simulink model "mekai_longitudinal_vehicle_starter"  (R2025b)
settings: Solver=ode45  StartTime=0.0  StopTime=simConfig.stopTime  RelTol=1e-3
undefined symbols (not defined in the file or in its folder): driver, params
settings Model: Creator=fabiofesta  LastModifiedBy=fabiofesta
settings DataIOCC: SaveFormat=StructureWithTime

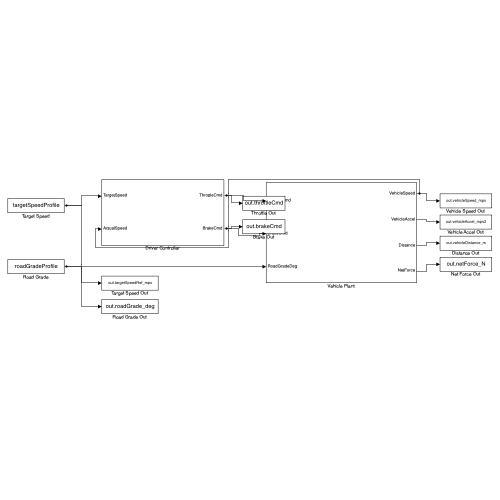
[thumbnail: Simulink's stored preview of the top-level diagram]
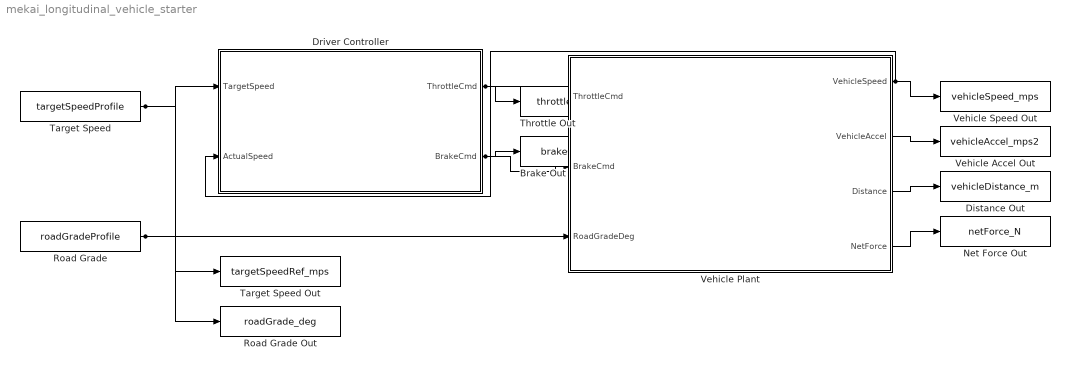
== system mekai_longitudinal_vehicle_starter ==
  Brake Out : ToWorkspace  VariableName=brakeCmd  SampleTime=-1
  Distance Out : ToWorkspace  VariableName=vehicleDistance_m  SampleTime=-1
  Driver Controller : Subsystem
  Net Force Out : ToWorkspace  VariableName=netForce_N  SampleTime=-1
  Road Grade : FromWorkspace  VariableName=roadGradeProfile
  Road Grade Out : ToWorkspace  VariableName=roadGrade_deg  SampleTime=-1
  Target Speed : FromWorkspace  VariableName=targetSpeedProfile
  Target Speed Out : ToWorkspace  VariableName=targetSpeedRef_mps  SampleTime=-1
  Throttle Out : ToWorkspace  VariableName=throttleCmd  SampleTime=-1
  Vehicle Accel Out : ToWorkspace  VariableName=vehicleAccel_mps2  SampleTime=-1
  Vehicle Plant : Subsystem
  Vehicle Speed Out : ToWorkspace  VariableName=vehicleSpeed_mps  SampleTime=-1
  wires:
  Target Speed/1 -> Driver Controller/1(TargetSpeed), Target Speed Out/1
  Road Grade/1 -> Vehicle Plant/3(RoadGradeDeg), Road Grade Out/1
  Vehicle Plant/1(VehicleSpeed) -> Driver Controller/2(ActualSpeed), Vehicle Speed Out/1
  Driver Controller/1(ThrottleCmd) -> Vehicle Plant/1(ThrottleCmd), Throttle Out/1
  Driver Controller/2(BrakeCmd) -> Vehicle Plant/2(BrakeCmd), Brake Out/1
  Vehicle Plant/2(VehicleAccel) -> Vehicle Accel Out/1
  Vehicle Plant/3(Distance) -> Distance Out/1
  Vehicle Plant/4(NetForce) -> Net Force Out/1

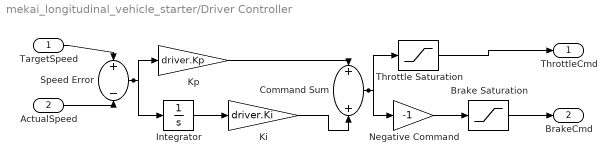
== system mekai_longitudinal_vehicle_starter/Driver Controller ==
  TargetSpeed : Inport
  ActualSpeed : Inport  Port=2
  Brake Saturation : Saturate  UpperLimit=1  LowerLimit=0
  Command Sum : Sum
  Integrator : Integrator
  Ki : Gain  Gain=driver.Ki
  Kp : Gain  Gain=driver.Kp
  Negative Command : Gain  Gain=-1
  Speed Error : Sum  Inputs=+-
  Throttle Saturation : Saturate  UpperLimit=1  LowerLimit=0
  ThrottleCmd : Outport
  BrakeCmd : Outport  Port=2
  wires:
  TargetSpeed/1 -> Speed Error/1
  ActualSpeed/1 -> Speed Error/2
  Speed Error/1 -> Kp/1, Integrator/1
  Integrator/1 -> Ki/1
  Kp/1 -> Command Sum/1
  Ki/1 -> Command Sum/2
  Command Sum/1 -> Throttle Saturation/1, Negative Command/1
  Negative Command/1 -> Brake Saturation/1
  Throttle Saturation/1 -> ThrottleCmd/1
  Brake Saturation/1 -> BrakeCmd/1

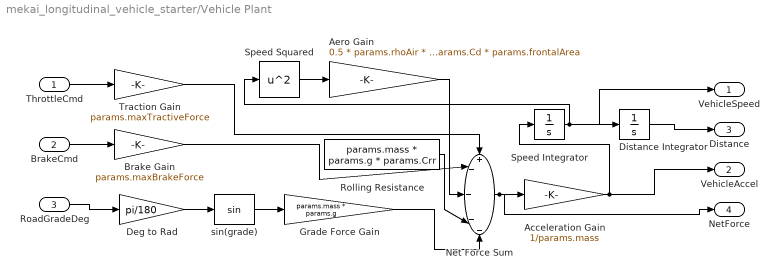
== system mekai_longitudinal_vehicle_starter/Vehicle Plant ==
  ThrottleCmd : Inport
  BrakeCmd : Inport  Port=2
  RoadGradeDeg : Inport  Port=3
  Acceleration Gain : Gain  Gain=1/params.mass
  Aero Gain : Gain  Gain=0.5 * params.rhoAir * params.Cd * params.frontalArea
  Brake Gain : Gain  Gain=params.maxBrakeForce
  Deg to Rad : Gain  Gain=pi/180
  Distance Integrator : Integrator  InitialCondition=params.initialDistance
  Grade Force Gain : Gain  Gain=params.mass * params.g
  Net Force Sum : Sum  Inputs=+----
  Rolling Resistance : Constant  Value=params.mass * params.g * params.Crr
  Speed Integrator : Integrator  InitialCondition=params.initialSpeed  LimitOutput=on  LowerSaturationLimit=0
  Speed Squared : Math  Operator=square
  Traction Gain : Gain  Gain=params.maxTractiveForce
  sin(grade) : Trigonometry
  VehicleSpeed : Outport
  VehicleAccel : Outport  Port=2
  Distance : Outport  Port=3
  NetForce : Outport  Port=4
  wires:
  ThrottleCmd/1 -> Traction Gain/1
  BrakeCmd/1 -> Brake Gain/1
  RoadGradeDeg/1 -> Deg to Rad/1
  Deg to Rad/1 -> sin(grade)/1
  sin(grade)/1 -> Grade Force Gain/1
  Speed Integrator/1 -> Speed Squared/1, Distance Integrator/1, VehicleSpeed/1
  Speed Squared/1 -> Aero Gain/1
  Traction Gain/1 -> Net Force Sum/1
  Brake Gain/1 -> Net Force Sum/2
  Aero Gain/1 -> Net Force Sum/3
  Rolling Resistance/1 -> Net Force Sum/4
  Grade Force Gain/1 -> Net Force Sum/5
  Net Force Sum/1 -> Acceleration Gain/1, NetForce/1
  Acceleration Gain/1 -> Speed Integrator/1, VehicleAccel/1
  Distance Integrator/1 -> Distance/1
